simulink model "Omnidirectional_robot_V3_pro1"  (R2020b)
settings: Solver=FixedStepAuto  StartTime=0.0  StopTime=20.0  FixedStep=1e-2  RelTol=1e-3
libraries: simulink x1
settings Model: Creator=Admin  LastModifiedBy=Admin

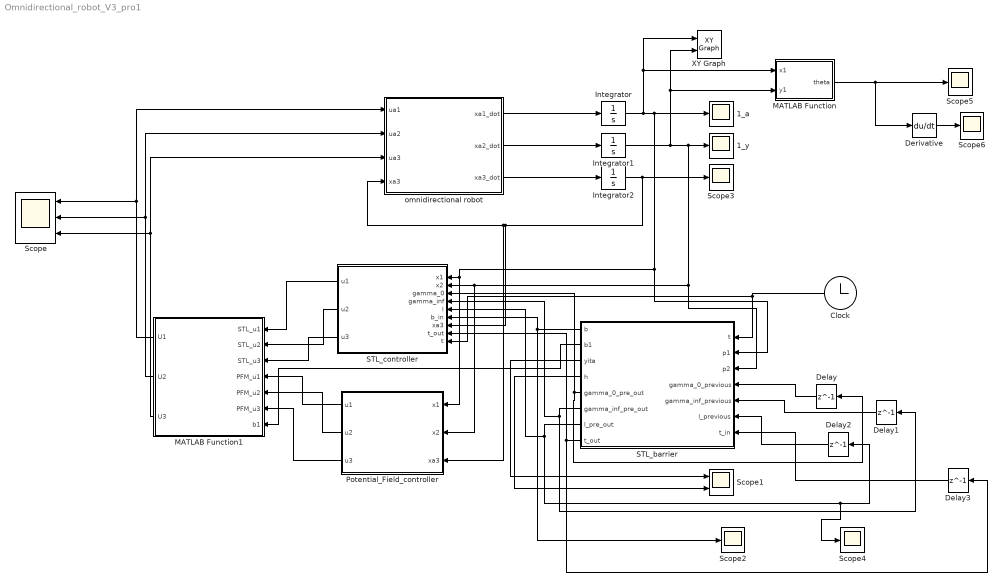
== system Omnidirectional_robot_V3_pro1 ==
  1_a : Scope
  1_y : Scope
  Clock : Clock
  Delay{,1..3} (4 alike) : Delay  DelayLength=1  InitialCondition=0
  Derivative : Derivative
  Integrator : Integrator
  Integrator1 : Integrator
  Integrator2 : Integrator
  MATLAB Function : MATLAB Function  TreatAsAtomicUnit=on
  MATLAB Function1 : MATLAB Function  TreatAsAtomicUnit=on
  Potential_Field_controller : MATLAB Function  TreatAsAtomicUnit=on
  "STL_barrier " : MATLAB Function  TreatAsAtomicUnit=on
  STL_controller : MATLAB Function  TreatAsAtomicUnit=on
  Scope : Scope  NumInputPorts=3
  Scope1 : Scope  NumInputPorts=2
  Scope{2..6} (5 alike) : Scope
  XY Graph : simulink/Sinks/XY Graph  xmin=-15  xmax=100  ymin=-15  ymax=100  st=0.01
  omnidirectional robot : MATLAB Function  TreatAsAtomicUnit=on
  wires:
  "STL_barrier "/1(b) -> Scope2/1, STL_controller/6(b_in)
  omnidirectional robot/1(xa1_dot) -> Integrator/1
  Derivative/1 -> Scope6/1
  MATLAB Function/1(theta) -> Derivative/1, Scope5/1
  Integrator1/1 -> MATLAB Function/2(y1), XY Graph/2, "STL_barrier "/3(p2), Potential_Field_controller/2(x2), STL_controller/2(x2), 1_y/1
  "STL_barrier "/3(yita) -> Scope1/1
  "STL_barrier "/4(h) -> Scope1/2
  Integrator2/1 -> Potential_Field_controller/3(xa3), omnidirectional robot/4(xa3), STL_controller/7(xa3), Scope3/1
  omnidirectional robot/3(xa3_dot) -> Integrator2/1
  Integrator/1 -> MATLAB Function/1(x1), XY Graph/1, "STL_barrier "/2(p1), Potential_Field_controller/1(x1), STL_controller/1(x1), 1_a/1
  Clock/1 -> STL_controller/9(t), "STL_barrier "/1(t)
  omnidirectional robot/2(xa2_dot) -> Integrator1/1
  STL_controller/1(u1) -> MATLAB Function1/1(STL_u1)
  STL_controller/2(u2) -> MATLAB Function1/2(STL_u2)
  STL_controller/3(u3) -> MATLAB Function1/3(STL_u3)
  Potential_Field_controller/1(u1) -> MATLAB Function1/4(PFM_u1)
  Potential_Field_controller/2(u2) -> MATLAB Function1/5(PFM_u2)
  Potential_Field_controller/3(u3) -> MATLAB Function1/6(PFM_u3)
  "STL_barrier "/2(b1) -> MATLAB Function1/7(b1)
  MATLAB Function1/1(U1) -> Scope/1, omnidirectional robot/1(ua1)
  MATLAB Function1/2(U2) -> Scope/2, omnidirectional robot/2(ua2)
  MATLAB Function1/3(U3) -> Scope/3, omnidirectional robot/3(ua3)
  "STL_barrier "/5(gamma_0_pre_out) -> Delay/1, STL_controller/3(gamma_0)
  "STL_barrier "/6(gamma_inf_pre_out) -> STL_controller/4(gamma_inf), Delay1/1
  "STL_barrier "/7(l_pre_out) -> STL_controller/5(l), Scope4/1, Delay2/1
  Delay/1 -> "STL_barrier "/4(gamma_0_previous)
  Delay1/1 -> "STL_barrier "/5(gamma_inf_previous)
  Delay2/1 -> "STL_barrier "/6(l_previous)
  "STL_barrier "/8(t_out) -> Delay3/1, STL_controller/8(t_out)
  Delay3/1 -> "STL_barrier "/7(t_in)

== matlab function Omnidirectional_robot_V3_pro1/STL_barrier  ==
  data: b output; b1 output; yita output; h output; t input; p1 input; p2 input; gamma_0_previous input; gamma_inf_previous input; l_previous input; gamma_0_pre_out output; gamma_inf_pre_out output; l_pre_out output; t_in input; t_out output
function [b,b1,yita,h,gamma_0_pre_out,gamma_inf_pre_out,l_pre_out, t_out] = fcn(t,p1,p2,gamma_0_previous,gamma_inf_previous,l_previous, t_in )
%% gamma_builder(x1_0, x2_0,x1_goal, x2_goal,R, t_star)
% (x1_0, x2_0) initial condition;
% (x1_goal, x2_goal) goal position;
%  R goal radius 
%  t_star important time
%%
d1=90;
d2=90;

obs1=50;
obs2=50;
x1_0 = 0; x2_0 = 0; x1_goal = d1; x2_goal = d2; R = 10; t_star =15;

yita=( gamma_0_previous - gamma_inf_previous )*exp(-l_previous*(t - t_in)) + gamma_inf_previous;
h=10-sqrt( (p1-d1)^2 + (p2-d2)^2 );
b= h - yita;


if t ==0
[gamma_0,gamma_inf,l] = gamma_builder(x1_0, x2_0,x1_goal, x2_goal,R, t_star);
yita=( gamma_0 - gamma_inf )*exp(-l*t) + gamma_inf;
h=10-sqrt( (p1-d1)^2 + (p2-d2)^2 );
b= h - yita;
gamma_0_pre_out = gamma_0;
gamma_inf_pre_out = gamma_inf;
l_pre_out = l;
t_out = 0;
else
    if b >=0
        gamma_0 = gamma_0_previous;
        gamma_inf = gamma_inf_previous;
        l = l_previous;
        yita=( gamma_0 - gamma_inf )*exp(-l*(t - t_in)) + gamma_inf;
        h=10-sqrt( (p1-d1)^2 + (p2-d2)^2 );
        b= h - yita;
        gamma_0_pre_out = gamma_0;
        gamma_inf_pre_out = gamma_inf;
        l_pre_out = l;
        t_out = t_in;
    else 
        t_out = t;
        [gamma_0,gamma_inf,l] = gamma_builder(p1, p2,x1_goal, x2_goal,R, t_star-t);
        yita=( gamma_0 - gamma_inf )*exp(-l*(t - t_out)) + gamma_inf;
        h=10-sqrt( (p1-d1)^2 + (p2-d2)^2 );
        b= h - yita; 
        gamma_0_pre_out = gamma_0;
        gamma_inf_pre_out = gamma_inf;
        l_pre_out = l;
    end
end

b1=sqrt( (p1-obs1)^2 + (p2-obs2)^2 )-16;

== matlab function Omnidirectional_robot_V3_pro1/omnidirectional robot ==
  data: ua1 input; xa1_dot output; ua2 input; ua3 input; xa3 input; xa2_dot output; xa3_dot output
function [xa1_dot,xa2_dot,xa3_dot]= fcn(ua1,ua2,ua3,xa3)

Li=0.2;
Bi=[0,cos(pi/6),-cos(pi/6);
    -1,sin(pi/6),sin(pi/6);
    Li,Li,Li;];

R1=[cos(xa3),-sin(xa3),0;
    sin(xa3),cos(xa3),0;
    0,0,1;];
R=0.02;

A=R1*inv(Bi')*R*[ua1;ua2;ua3];
xa1_dot=A(1,1);
xa2_dot=A(2,1);
xa3_dot=A(3,1);

== matlab function Omnidirectional_robot_V3_pro1/STL_controller ==
  data: x1 input; x2 input; gamma_0 input; gamma_inf input; l input; b_in input; u1 output; xa3 input; t_out input; u2 output; u3 output; t input
function [u1,u2,u3]= fcn(x1, x2,gamma_0,gamma_inf,l, b_in, xa3,t_out,t)
coder.extrinsic('quadoptimizer');
%coder.extrinsic('save');
%%
d1=90; d2=90;
% x1_0 = 0; x2_0 = 0; x1_goal = d1; x2_goal = d2; R = 10; t_star =15;
% [gamma_0,gamma_inf,l] = gamma_builder(x1_0, x2_0,x1_goal, x2_goal,R, t_star);
yita=( gamma_0 - gamma_inf )*exp(-l*t) + gamma_inf;
h=10-sqrt( (x1-d1)^2 + (x2-d2)^2 );
b= h - yita;
%%
partial_b=(1/2)*((x1-d1)^2+(x2-d2)^2)^(-1/2);
partial_b_x=[-2*partial_b*(x1-d1),-2*partial_b*(x2-d2),0];


Li=0.2;
Bi=[0,cos(pi/6),-cos(pi/6);
    -1,sin(pi/6),sin(pi/6);
    Li,Li,Li;];

R1=[cos(xa3),-sin(xa3),0;
    sin(xa3),cos(xa3),0;
    0,0,1;];
R=0.02;

gx=R1*inv(Bi')*R;

A=partial_b_x*gx;
% A=[A;-gx];

H=[1,0,0;0,1,0;0,0,1];
%H=[1];
partial_b_t = l * ( gamma_0 - gamma_inf ) * exp(-l*(t-t_out));
b= 0.1* (b_in-0) + partial_b_t ;
% b=[b;5000;5000;5000]


u1=0;u2=0;u3=0;
U=quadoptimizer(H,b,A);

%U=quadprod(H,[],-A,b);

u1=U(1,1);
u2=U(2,1);
u3=U(3,1);

== matlab function Omnidirectional_robot_V3_pro1/MATLAB Function ==
  data: x1 input; theta output; y1 input
function theta = fcn(x1, y1)
theta=atan2(y1,x1);

== matlab function Omnidirectional_robot_V3_pro1/Potential_Field_controller ==
  data: x1 input; x2 input; u1 output; xa3 input; u2 output; u3 output
function [u1,u2,u3] = fcn(x1, x2, xa3)
coder.extrinsic('Calculate_gradient');
coder.extrinsic('PVF_optimizer');
coder.extrinsic('add_random');
A1=[-1,0;0,-1];
F=[180,180];
distance=sqrt((x1-90)^2+(x2-90)^2);
gradient_x=0;gradient_y=0;
[gradient_x,gradient_y]=Calculate_gradient(x1,x2,A1,F,50,50,20);
% gradient_x=Gradient(1,1);
% gradient_y=Gradient(1,2);
gradient_z=0;
Gradient_all=[gradient_x;gradient_y;gradient_z];

Li=0.2;
Bi=[0,cos(pi/6),-cos(pi/6);
    -1,sin(pi/6),sin(pi/6);
    Li,Li,Li;];

R1=[cos(xa3),-sin(xa3),0;
    sin(xa3),cos(xa3),0;
    0,0,1;];
R=0.02;
gx=R1*inv(Bi')*R;
A=Gradient_all'*gx;

%H=[1];
%H=[1,0;0,1];
%H=[0,0,0;0,0,0;0,0,0];
% H=[1,0,0;0,1,0;0,0,1];
 H=(1/2)*gx'*gx;
b=[0];
F=[-2*gx'*50*Gradient_all];
%=[];
u1=0;u2=0;u3=0;
U=PVF_optimizer(H,b,A,F,distance,gradient_x,gradient_y);

u1=U(1,1);
u2=U(2,1);
u3=U(3,1);

== matlab function Omnidirectional_robot_V3_pro1/MATLAB Function1 ==
  data: STL_u1 input; U1 output; STL_u2 input; STL_u3 input; PFM_u1 input; PFM_u2 input; PFM_u3 input; b1 input; U2 output; U3 output
function [U1,U2,U3] = fcn(STL_u1,STL_u2,STL_u3,PFM_u1,PFM_u2,PFM_u3,b1)
U_goal=[STL_u1;STL_u2;STL_u3];
U_obs=[PFM_u1;PFM_u2;PFM_u3];
k=0.15;
lambda=1-exp(-k*max(b1,0));
U=lambda*U_goal+(1-lambda)*U_obs;
U1=0;U2=0;U3=0;
U1=U(1,1);
U2=U(2,1);
U3=U(3,1);
